simulink model "MySuspKnC_RTW"  (Simulink 9.3)
settings: Solver=ode1  StartTime=0.0  StopTime=inf  FixedStep=0.001  RelTol=1e-3
PreLoadFcn:
  | vehicle = 'Car'; if ~length(which('cmself')), cmenv; end
  | MySuspKnC_RTW_bus
InitFcn:
  | vehicle = 'Car'; if ~length(which('cmself')), cmenv; end
  | MySuspKnC_RTW_bus
Description:
  | CarMaker Plug-in Model Target
settings Model: Creator=ml  LastModifiedBy=ml
settings DataIOCC: SaveFormat=Dataset  SignalLoggingSaveFormat=Dataset  ReturnWorkspaceOutputs=on
settings OptimizationCC: LifeSpan=auto
settings DebuggingCC: UnderspecifiedInitializationDetection=Simplified  MergeDetectMultiDrivingBlocksExec=error  FcnCallInpInsideContextMsg=error  SFUnexpectedBacktrackingDiag=error  SFNoUnconditionalDefaultTransitionDiag=error  SFExecutionAtInitializationDiag=warning  ArithmeticOperatorsInVariantConditions=error
settings HardwareCC: ProdBitPerPointer=64  ProdBitPerSizeT=64  ProdBitPerPtrDiffT=64  ProdLargestAtomicFloat=Float  ProdIntDivRoundTo=Zero  ProdEndianess=LittleEndian  ProdWordSize=64  ProdHWDeviceType=Intel->x86-64 (Windows64)
settings ModelReferenceCC: PropagateSignalLabelsOutOfModel=on
settings SFSimCC: SimUseLocalCustomCode=on
settings RTWCC: SystemTargetFile=CarMaker.tlc  TemplateMakefile=CarMaker_unix-win64.tmf  Description=CarMaker Plug-in Model Target  RTWUseLocalCustomCode=on
settings CodeAppCC: MaxIdLength=127  StateflowObjectComments=off
settings STFCustomTargetCC: TargetLangStandard=C99 (ISO)  CombineOutputUpdateFcns=on  MultiInstanceERTCode=on  CodeInterfacePackaging=Reusable function  GRTInterface=off  GenerateAllocFcn=on  SystemTargetFile=CarMaker.tlc
settings GRTTargetCC: TargetLangStandard=C99 (ISO)  ParMdlRefBuildCompliant=off  CompOptLevelCompliant=off  ConcurrentExecutionCompliant=off  CombineOutputUpdateFcns=on  MatFileLogging=off  MultiInstanceERTCode=on  CodeInterfacePackaging=Reusable function  CPPClassGenCompliant=off  GRTInterface=off  GenerateAllocFcn=on  UseToolchainInfoCompliant=off  RTWCAPISignals=on  RTWCAPIParams=on
settings CustomProperty: DataType=string
settings EnumStrPairs: String=Car
settings ConfigComp: CovMetricSettings=dwe  CovHtmlReporting=off  CovSaveCumulativeToWorkspaceVar=off  CovSaveSingleToWorkspaceVar=off  CovExternalEMLEnable=on

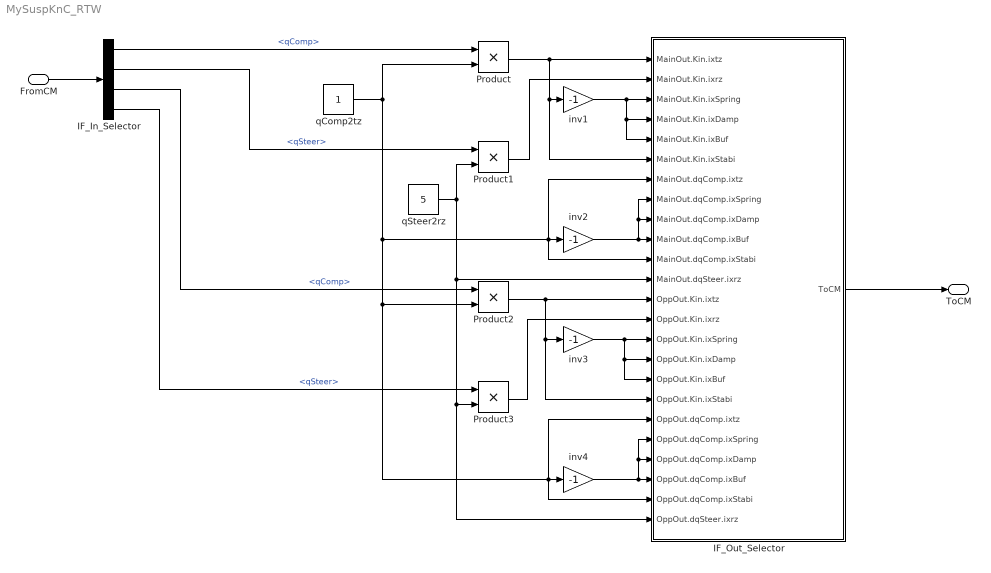
== system MySuspKnC_RTW ==
  FromCM : Inport  OutDataTypeStr=Bus: cmSuspKnCIn
  IF_In_Selector : BusSelector  OutputSignals=MainIn.qComp,MainIn.qSteer,OppIn.qComp,OppIn.qSteer
  IF_Out_Selector : Subsystem  mask(Signal Selection){}
      mask help: Signal Selection Block
      settings: OpenFcn=cmSignalSelect('SignalSelection_CB',gcb)
  Product{,1..3} (4 alike) : Product
  inv{1..4} (4 alike) : Gain  Gain=-1
  qComp2tz : Constant
  qSteer2rz : Constant  Value=5
  ToCM : Outport  OutDataTypeStr=Bus: cmSuspKnCOut
  wires:
  FromCM/1 -> IF_In_Selector/1
  IF_Out_Selector/1(ToCM) -> ToCM/1
  qSteer2rz/1 -> Product1/2, IF_Out_Selector/12(MainOut.dqSteer.ixrz), IF_Out_Selector/24(OppOut.dqSteer.ixrz), Product3/2
  IF_In_Selector/1 -> Product/1  "<qComp>"
  IF_In_Selector/2 -> Product1/1  "<qSteer>"
  qComp2tz/1 -> Product/2, IF_Out_Selector/7(MainOut.dqComp.ixtz), inv2/1, IF_Out_Selector/11(MainOut.dqComp.ixStabi), IF_Out_Selector/19(OppOut.dqComp.ixtz), IF_Out_Selector/23(OppOut.dqComp.ixStabi), inv4/1, Product2/2
  Product/1 -> IF_Out_Selector/6(MainOut.Kin.ixStabi), inv1/1, IF_Out_Selector/1(MainOut.Kin.ixtz)
  Product1/1 -> IF_Out_Selector/2(MainOut.Kin.ixrz)
  inv2/1 -> IF_Out_Selector/9(MainOut.dqComp.ixDamp), IF_Out_Selector/8(MainOut.dqComp.ixSpring), IF_Out_Selector/10(MainOut.dqComp.ixBuf)
  inv1/1 -> IF_Out_Selector/3(MainOut.Kin.ixSpring), IF_Out_Selector/4(MainOut.Kin.ixDamp), IF_Out_Selector/5(MainOut.Kin.ixBuf)
  IF_In_Selector/3 -> Product2/1  "<qComp>"
  IF_In_Selector/4 -> Product3/1  "<qSteer>"
  inv3/1 -> IF_Out_Selector/17(OppOut.Kin.ixBuf), IF_Out_Selector/16(OppOut.Kin.ixDamp), IF_Out_Selector/15(OppOut.Kin.ixSpring)
  Product2/1 -> IF_Out_Selector/18(OppOut.Kin.ixStabi), inv3/1, IF_Out_Selector/13(OppOut.Kin.ixtz)
  Product3/1 -> IF_Out_Selector/14(OppOut.Kin.ixrz)
  inv4/1 -> IF_Out_Selector/20(OppOut.dqComp.ixSpring), IF_Out_Selector/21(OppOut.dqComp.ixDamp), IF_Out_Selector/22(OppOut.dqComp.ixBuf)

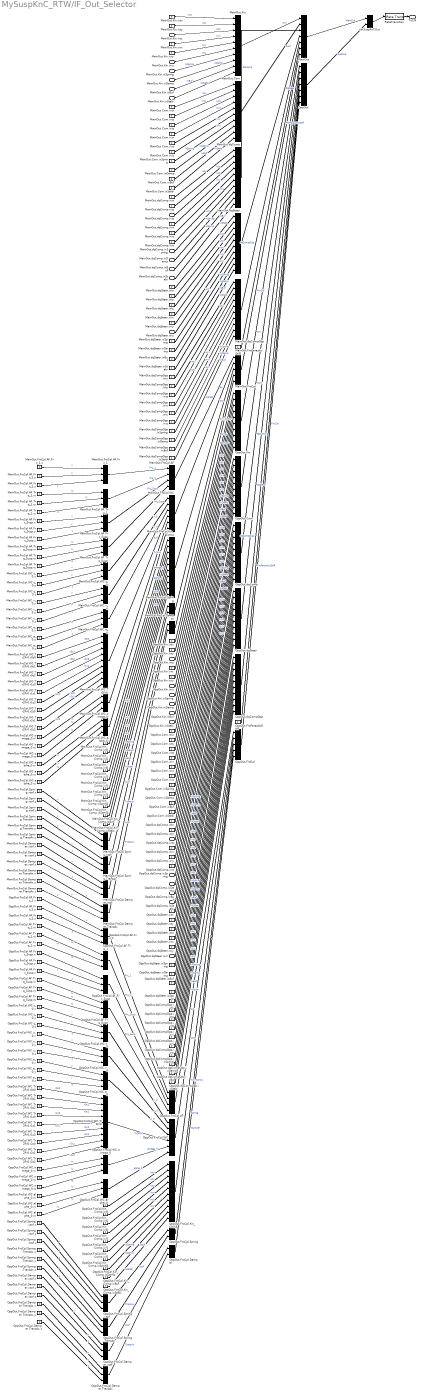
== system MySuspKnC_RTW/IF_Out_Selector ==
  MainOut.Kin.ixtz : Inport
  MainOut.Kin.ixrz : Inport  Port=2
  MainOut.Kin.ixSpring : Inport  Port=3
  MainOut.Kin.ixDamp : Inport  Port=4
  MainOut.Kin.ixBuf : Inport  Port=5
  MainOut.Kin.ixStabi : Inport  Port=6
  MainOut.dqComp.ixtz : Inport  Port=7
  MainOut.dqComp.ixSpring : Inport  Port=8
  MainOut.dqComp.ixDamp : Inport  Port=9
  MainOut.dqComp.ixBuf : Inport  Port=10
  MainOut.dqComp.ixStabi : Inport  Port=11
  MainOut.dqSteer.ixrz : Inport  Port=12
  OppOut.Kin.ixtz : Inport  Port=13
  OppOut.Kin.ixrz : Inport  Port=14
  OppOut.Kin.ixSpring : Inport  Port=15
  OppOut.Kin.ixDamp : Inport  Port=16
  OppOut.Kin.ixBuf : Inport  Port=17
  OppOut.Kin.ixStabi : Inport  Port=18
  OppOut.dqComp.ixtz : Inport  Port=19
  OppOut.dqComp.ixSpring : Inport  Port=20
  OppOut.dqComp.ixDamp : Inport  Port=21
  OppOut.dqComp.ixBuf : Inport  Port=22
  OppOut.dqComp.ixStabi : Inport  Port=23
  OppOut.dqSteer.ixrz : Inport  Port=24
  MainOut : BusCreator  Inputs=7
  MainOut.Com : BusCreator  Inputs=10
  MainOut.Com.ixBuf : Constant  Value=0
  MainOut.Com.ixDamp : Constant  Value=0
  MainOut.Com.ixSpring : Constant  Value=0
  MainOut.Com.ixStabi : Constant  Value=0
  MainOut.Com.ixrx : Constant  Value=0
  MainOut.Com.ixry : Constant  Value=0
  MainOut.Com.ixrz : Constant  Value=0
  MainOut.Com.ixtx : Constant  Value=0
  MainOut.Com.ixty : Constant  Value=0
  MainOut.Com.ixtz : Constant  Value=0
  MainOut.FrcCpl : BusCreator  Inputs=5
  MainOut.FrcCpl.AF : BusCreator  Inputs=4
  MainOut.FrcCpl.AF.Frc_1 : BusCreator  Inputs=3
  MainOut.FrcCpl.AF.Frc_1.x : Constant  Value=0
  MainOut.FrcCpl.AF.Frc_1.y : Constant  Value=0
  MainOut.FrcCpl.AF.Frc_1.z : Constant  Value=0
  MainOut.FrcCpl.AF.Frc_Susp : BusCreator  Inputs=3
  MainOut.FrcCpl.AF.Frc_Susp.x : Constant  Value=0
  MainOut.FrcCpl.AF.Frc_Susp.y : Constant  Value=0
  MainOut.FrcCpl.AF.Frc_Susp.z : Constant  Value=0
  MainOut.FrcCpl.AF.Trq_1 : BusCreator  Inputs=3
  MainOut.FrcCpl.AF.Trq_1.rx : Constant  Value=0
  MainOut.FrcCpl.AF.Trq_1.ry : Constant  Value=0
  MainOut.FrcCpl.AF.Trq_1.rz : Constant  Value=0
  MainOut.FrcCpl.AF.Trq_Susp : BusCreator  Inputs=3
  MainOut.FrcCpl.AF.Trq_Susp.rx : Constant  Value=0
  MainOut.FrcCpl.AF.Trq_Susp.ry : Constant  Value=0
  MainOut.FrcCpl.AF.Trq_Susp.rz : Constant  Value=0
  MainOut.FrcCpl.Damper : BusCreator  Inputs=2
  MainOut.FrcCpl.Damper.TransAx : BusCreator  Inputs=3
  MainOut.FrcCpl.Damper.TransAx.x : Constant  Value=0
  MainOut.FrcCpl.Damper.TransAx.y : Constant  Value=0
  MainOut.FrcCpl.Damper.TransAx.z : Constant  Value=0
  MainOut.FrcCpl.Damper.xtof : BusCreator  Inputs=3
  MainOut.FrcCpl.Damper.xtof.x : Constant  Value=0
  MainOut.FrcCpl.Damper.xtof.y : Constant  Value=0
  MainOut.FrcCpl.Damper.xtof.z : Constant  Value=0
  MainOut.FrcCpl.Kin_Comp : BusCreator  Inputs=10
  MainOut.FrcCpl.Kin_Comp.ixBuf : Constant  Value=0
  MainOut.FrcCpl.Kin_Comp.ixDamp : Constant  Value=0
  MainOut.FrcCpl.Kin_Comp.ixSpring : Constant  Value=0
  MainOut.FrcCpl.Kin_Comp.ixStabi : Constant  Value=0
  MainOut.FrcCpl.Kin_Comp.ixrx : Constant  Value=0
  MainOut.FrcCpl.Kin_Comp.ixry : Constant  Value=0
  MainOut.FrcCpl.Kin_Comp.ixrz : Constant  Value=0
  MainOut.FrcCpl.Kin_Comp.ixtx : Constant  Value=0
  MainOut.FrcCpl.Kin_Comp.ixty : Constant  Value=0
  MainOut.FrcCpl.Kin_Comp.ixtz : Constant  Value=0
  MainOut.FrcCpl.Spring : BusCreator  Inputs=2
  MainOut.FrcCpl.Spring.TransAx : BusCreator  Inputs=3
  MainOut.FrcCpl.Spring.TransAx.x : Constant  Value=0
  MainOut.FrcCpl.Spring.TransAx.y : Constant  Value=0
  MainOut.FrcCpl.Spring.TransAx.z : Constant  Value=0
  MainOut.FrcCpl.Spring.xtof : BusCreator  Inputs=3
  MainOut.FrcCpl.Spring.xtof.x : Constant  Value=0
  MainOut.FrcCpl.Spring.xtof.y : Constant  Value=0
  MainOut.FrcCpl.Spring.xtof.z : Constant  Value=0
  MainOut.FrcCpl.WC : BusCreator  Inputs=6
  MainOut.FrcCpl.WC.Tr2Fr0 : BusCreator  Inputs=9
  MainOut.FrcCpl.WC.Tr2Fr0.r0c0 : Constant  Value=0
  MainOut.FrcCpl.WC.Tr2Fr0.r0c1 : Constant  Value=0
  MainOut.FrcCpl.WC.Tr2Fr0.r0c2 : Constant  Value=0
  MainOut.FrcCpl.WC.Tr2Fr0.r1c0 : Constant  Value=0
  MainOut.FrcCpl.WC.Tr2Fr0.r1c1 : Constant  Value=0
  MainOut.FrcCpl.WC.Tr2Fr0.r1c2 : Constant  Value=0
  MainOut.FrcCpl.WC.Tr2Fr0.r2c0 : Constant  Value=0
  MainOut.FrcCpl.WC.Tr2Fr0.r2c1 : Constant  Value=0
  MainOut.FrcCpl.WC.Tr2Fr0.r2c2 : Constant  Value=0
  MainOut.FrcCpl.WC.a_0 : BusCreator  Inputs=3
  MainOut.FrcCpl.WC.a_0.x : Constant  Value=0
  MainOut.FrcCpl.WC.a_0.y : Constant  Value=0
  MainOut.FrcCpl.WC.a_0.z : Constant  Value=0
  MainOut.FrcCpl.WC.alpha_0 : BusCreator  Inputs=3
  MainOut.FrcCpl.WC.alpha_0.rx : Constant  Value=0
  MainOut.FrcCpl.WC.alpha_0.ry : Constant  Value=0
  MainOut.FrcCpl.WC.alpha_0.rz : Constant  Value=0
  MainOut.FrcCpl.WC.omega_0 : BusCreator  Inputs=3
  MainOut.FrcCpl.WC.omega_0.rx : Constant  Value=0
  MainOut.FrcCpl.WC.omega_0.ry : Constant  Value=0
  MainOut.FrcCpl.WC.omega_0.rz : Constant  Value=0
  MainOut.FrcCpl.WC.t_0 : BusCreator  Inputs=3
  MainOut.FrcCpl.WC.t_0.x : Constant  Value=0
  MainOut.FrcCpl.WC.t_0.y : Constant  Value=0
  MainOut.FrcCpl.WC.t_0.z : Constant  Value=0
  MainOut.FrcCpl.WC.v_0 : BusCreator  Inputs=3
  MainOut.FrcCpl.WC.v_0.x : Constant  Value=0
  MainOut.FrcCpl.WC.v_0.y : Constant  Value=0
  MainOut.FrcCpl.WC.v_0.z : Constant  Value=0
  MainOut.FrcParasiticStiff : Constant  Value=0
  MainOut.Kin : BusCreator  Inputs=10
  MainOut.Kin.ixrx : Constant  Value=0
  MainOut.Kin.ixry : Constant  Value=0
  MainOut.Kin.ixtx : Constant  Value=0
  MainOut.Kin.ixty : Constant  Value=0
  MainOut.dqComp : BusCreator  Inputs=10
  MainOut.dqComp.ixrx : Constant  Value=0
  MainOut.dqComp.ixry : Constant  Value=0
  MainOut.dqComp.ixrz : Constant  Value=0
  MainOut.dqComp.ixtx : Constant  Value=0
  MainOut.dqComp.ixty : Constant  Value=0
  MainOut.dqCompOpp : BusCreator  Inputs=10
  MainOut.dqCompOpp.ixBuf : Constant  Value=0
  MainOut.dqCompOpp.ixDamp : Constant  Value=0
  MainOut.dqCompOpp.ixSpring : Constant  Value=0
  MainOut.dqCompOpp.ixStabi : Constant  Value=0
  MainOut.dqCompOpp.ixrx : Constant  Value=0
  MainOut.dqCompOpp.ixry : Constant  Value=0
  MainOut.dqCompOpp.ixrz : Constant  Value=0
  MainOut.dqCompOpp.ixtx : Constant  Value=0
  MainOut.dqCompOpp.ixty : Constant  Value=0
  MainOut.dqCompOpp.ixtz : Constant  Value=0
  MainOut.dqSteer : BusCreator  Inputs=10
  MainOut.dqSteer.ixBuf : Constant  Value=0
  MainOut.dqSteer.ixDamp : Constant  Value=0
  MainOut.dqSteer.ixSpring : Constant  Value=0
  MainOut.dqSteer.ixStabi : Constant  Value=0
  MainOut.dqSteer.ixrx : Constant  Value=0
  MainOut.dqSteer.ixry : Constant  Value=0
  MainOut.dqSteer.ixtx : Constant  Value=0
  MainOut.dqSteer.ixty : Constant  Value=0
  MainOut.dqSteer.ixtz : Constant  Value=0
  OppOut : BusCreator  Inputs=7
  OppOut.Com : BusCreator  Inputs=10
  OppOut.Com.ixBuf : Constant  Value=0
  OppOut.Com.ixDamp : Constant  Value=0
  OppOut.Com.ixSpring : Constant  Value=0
  OppOut.Com.ixStabi : Constant  Value=0
  OppOut.Com.ixrx : Constant  Value=0
  OppOut.Com.ixry : Constant  Value=0
  OppOut.Com.ixrz : Constant  Value=0
  OppOut.Com.ixtx : Constant  Value=0
  OppOut.Com.ixty : Constant  Value=0
  OppOut.Com.ixtz : Constant  Value=0
  OppOut.FrcCpl : BusCreator  Inputs=5
  OppOut.FrcCpl.AF : BusCreator  Inputs=4
  OppOut.FrcCpl.AF.Frc_1 : BusCreator  Inputs=3
  OppOut.FrcCpl.AF.Frc_1.x : Constant  Value=0
  OppOut.FrcCpl.AF.Frc_1.y : Constant  Value=0
  OppOut.FrcCpl.AF.Frc_1.z : Constant  Value=0
  OppOut.FrcCpl.AF.Frc_Susp : BusCreator  Inputs=3
  OppOut.FrcCpl.AF.Frc_Susp.x : Constant  Value=0
  OppOut.FrcCpl.AF.Frc_Susp.y : Constant  Value=0
  OppOut.FrcCpl.AF.Frc_Susp.z : Constant  Value=0
  OppOut.FrcCpl.AF.Trq_1 : BusCreator  Inputs=3
  OppOut.FrcCpl.AF.Trq_1.rx : Constant  Value=0
  OppOut.FrcCpl.AF.Trq_1.ry : Constant  Value=0
  OppOut.FrcCpl.AF.Trq_1.rz : Constant  Value=0
  OppOut.FrcCpl.AF.Trq_Susp : BusCreator  Inputs=3
  OppOut.FrcCpl.AF.Trq_Susp.rx : Constant  Value=0
  OppOut.FrcCpl.AF.Trq_Susp.ry : Constant  Value=0
  OppOut.FrcCpl.AF.Trq_Susp.rz : Constant  Value=0
  OppOut.FrcCpl.Damper : BusCreator  Inputs=2
  OppOut.FrcCpl.Damper.TransAx : BusCreator  Inputs=3
  OppOut.FrcCpl.Damper.TransAx.x : Constant  Value=0
  OppOut.FrcCpl.Damper.TransAx.y : Constant  Value=0
  OppOut.FrcCpl.Damper.TransAx.z : Constant  Value=0
  OppOut.FrcCpl.Damper.xtof : BusCreator  Inputs=3
  OppOut.FrcCpl.Damper.xtof.x : Constant  Value=0
  OppOut.FrcCpl.Damper.xtof.y : Constant  Value=0
  OppOut.FrcCpl.Damper.xtof.z : Constant  Value=0
  OppOut.FrcCpl.Kin_Comp : BusCreator  Inputs=10
  OppOut.FrcCpl.Kin_Comp.ixBuf : Constant  Value=0
  OppOut.FrcCpl.Kin_Comp.ixDamp : Constant  Value=0
  OppOut.FrcCpl.Kin_Comp.ixSpring : Constant  Value=0
  OppOut.FrcCpl.Kin_Comp.ixStabi : Constant  Value=0
  OppOut.FrcCpl.Kin_Comp.ixrx : Constant  Value=0
  OppOut.FrcCpl.Kin_Comp.ixry : Constant  Value=0
  OppOut.FrcCpl.Kin_Comp.ixrz : Constant  Value=0
  OppOut.FrcCpl.Kin_Comp.ixtx : Constant  Value=0
  OppOut.FrcCpl.Kin_Comp.ixty : Constant  Value=0
  OppOut.FrcCpl.Kin_Comp.ixtz : Constant  Value=0
  OppOut.FrcCpl.Spring : BusCreator  Inputs=2
  OppOut.FrcCpl.Spring.TransAx : BusCreator  Inputs=3
  OppOut.FrcCpl.Spring.TransAx.x : Constant  Value=0
  OppOut.FrcCpl.Spring.TransAx.y : Constant  Value=0
  OppOut.FrcCpl.Spring.TransAx.z : Constant  Value=0
  OppOut.FrcCpl.Spring.xtof : BusCreator  Inputs=3
  OppOut.FrcCpl.Spring.xtof.x : Constant  Value=0
  OppOut.FrcCpl.Spring.xtof.y : Constant  Value=0
  OppOut.FrcCpl.Spring.xtof.z : Constant  Value=0
  OppOut.FrcCpl.WC : BusCreator  Inputs=6
  OppOut.FrcCpl.WC.Tr2Fr0 : BusCreator  Inputs=9
  OppOut.FrcCpl.WC.Tr2Fr0.r0c0 : Constant  Value=0
  OppOut.FrcCpl.WC.Tr2Fr0.r0c1 : Constant  Value=0
  OppOut.FrcCpl.WC.Tr2Fr0.r0c2 : Constant  Value=0
  OppOut.FrcCpl.WC.Tr2Fr0.r1c0 : Constant  Value=0
  OppOut.FrcCpl.WC.Tr2Fr0.r1c1 : Constant  Value=0
  OppOut.FrcCpl.WC.Tr2Fr0.r1c2 : Constant  Value=0
  OppOut.FrcCpl.WC.Tr2Fr0.r2c0 : Constant  Value=0
  OppOut.FrcCpl.WC.Tr2Fr0.r2c1 : Constant  Value=0
  OppOut.FrcCpl.WC.Tr2Fr0.r2c2 : Constant  Value=0
  OppOut.FrcCpl.WC.a_0 : BusCreator  Inputs=3
  OppOut.FrcCpl.WC.a_0.x : Constant  Value=0
  OppOut.FrcCpl.WC.a_0.y : Constant  Value=0
  OppOut.FrcCpl.WC.a_0.z : Constant  Value=0
  OppOut.FrcCpl.WC.alpha_0 : BusCreator  Inputs=3
  OppOut.FrcCpl.WC.alpha_0.rx : Constant  Value=0
  OppOut.FrcCpl.WC.alpha_0.ry : Constant  Value=0
  OppOut.FrcCpl.WC.alpha_0.rz : Constant  Value=0
  OppOut.FrcCpl.WC.omega_0 : BusCreator  Inputs=3
  OppOut.FrcCpl.WC.omega_0.rx : Constant  Value=0
  OppOut.FrcCpl.WC.omega_0.ry : Constant  Value=0
  OppOut.FrcCpl.WC.omega_0.rz : Constant  Value=0
  OppOut.FrcCpl.WC.t_0 : BusCreator  Inputs=3
  OppOut.FrcCpl.WC.t_0.x : Constant  Value=0
  OppOut.FrcCpl.WC.t_0.y : Constant  Value=0
  OppOut.FrcCpl.WC.t_0.z : Constant  Value=0
  OppOut.FrcCpl.WC.v_0 : BusCreator  Inputs=3
  OppOut.FrcCpl.WC.v_0.x : Constant  Value=0
  OppOut.FrcCpl.WC.v_0.y : Constant  Value=0
  OppOut.FrcCpl.WC.v_0.z : Constant  Value=0
  OppOut.FrcParasiticStiff : Constant  Value=0
  OppOut.Kin : BusCreator  Inputs=10
  OppOut.Kin.ixrx : Constant  Value=0
  OppOut.Kin.ixry : Constant  Value=0
  OppOut.Kin.ixtx : Constant  Value=0
  OppOut.Kin.ixty : Constant  Value=0
  OppOut.dqComp : BusCreator  Inputs=10
  OppOut.dqComp.ixrx : Constant  Value=0
  OppOut.dqComp.ixry : Constant  Value=0
  OppOut.dqComp.ixrz : Constant  Value=0
  OppOut.dqComp.ixtx : Constant  Value=0
  OppOut.dqComp.ixty : Constant  Value=0
  OppOut.dqCompOpp : BusCreator  Inputs=10
  OppOut.dqCompOpp.ixBuf : Constant  Value=0
  OppOut.dqCompOpp.ixDamp : Constant  Value=0
  OppOut.dqCompOpp.ixSpring : Constant  Value=0
  OppOut.dqCompOpp.ixStabi : Constant  Value=0
  OppOut.dqCompOpp.ixrx : Constant  Value=0
  OppOut.dqCompOpp.ixry : Constant  Value=0
  OppOut.dqCompOpp.ixrz : Constant  Value=0
  OppOut.dqCompOpp.ixtx : Constant  Value=0
  OppOut.dqCompOpp.ixty : Constant  Value=0
  OppOut.dqCompOpp.ixtz : Constant  Value=0
  OppOut.dqSteer : BusCreator  Inputs=10
  OppOut.dqSteer.ixBuf : Constant  Value=0
  OppOut.dqSteer.ixDamp : Constant  Value=0
  OppOut.dqSteer.ixSpring : Constant  Value=0
  OppOut.dqSteer.ixStabi : Constant  Value=0
  OppOut.dqSteer.ixrx : Constant  Value=0
  OppOut.dqSteer.ixry : Constant  Value=0
  OppOut.dqSteer.ixtx : Constant  Value=0
  OppOut.dqSteer.ixty : Constant  Value=0
  OppOut.dqSteer.ixtz : Constant  Value=0
  RateTransition : RateTransition  OutPortSampleTime=str2num(get_param(bdroot,'FixedStep'))
  cmSuspKnCOut : BusCreator  Inputs=2
  ToCM : Outport
  wires:
  RateTransition/1 -> ToCM/1
  cmSuspKnCOut/1 -> RateTransition/1
  MainOut/1 -> cmSuspKnCOut/1  "MainOut"
  MainOut.Kin/1 -> MainOut/1  "Kin"
  MainOut.Com/1 -> MainOut/2  "Com"
  MainOut.Com.ixtx/1 -> MainOut.Com/1  "ixtx"
  MainOut.Com.ixty/1 -> MainOut.Com/2  "ixty"
  MainOut.Com.ixtz/1 -> MainOut.Com/3  "ixtz"
  MainOut.Com.ixrx/1 -> MainOut.Com/4  "ixrx"
  MainOut.Com.ixry/1 -> MainOut.Com/5  "ixry"
  MainOut.Com.ixrz/1 -> MainOut.Com/6  "ixrz"
  MainOut.Com.ixSpring/1 -> MainOut.Com/7  "ixSpring"
  MainOut.Com.ixDamp/1 -> MainOut.Com/8  "ixDamp"
  MainOut.Com.ixBuf/1 -> MainOut.Com/9  "ixBuf"
  MainOut.Com.ixStabi/1 -> MainOut.Com/10  "ixStabi"
  MainOut.dqComp/1 -> MainOut/3  "dqComp"
  MainOut.dqComp.ixtx/1 -> MainOut.dqComp/1  "ixtx"
  MainOut.dqComp.ixty/1 -> MainOut.dqComp/2  "ixty"
  MainOut.dqComp.ixrx/1 -> MainOut.dqComp/4  "ixrx"
  MainOut.dqComp.ixry/1 -> MainOut.dqComp/5  "ixry"
  MainOut.dqComp.ixrz/1 -> MainOut.dqComp/6  "ixrz"
  MainOut.dqSteer/1 -> MainOut/4  "dqSteer"
  MainOut.dqSteer.ixtx/1 -> MainOut.dqSteer/1  "ixtx"
  MainOut.dqSteer.ixty/1 -> MainOut.dqSteer/2  "ixty"
  MainOut.dqSteer.ixtz/1 -> MainOut.dqSteer/3  "ixtz"
  MainOut.dqSteer.ixrx/1 -> MainOut.dqSteer/4  "ixrx"
  MainOut.dqSteer.ixry/1 -> MainOut.dqSteer/5  "ixry"
  MainOut.dqSteer.ixSpring/1 -> MainOut.dqSteer/7  "ixSpring"
  MainOut.dqSteer.ixDamp/1 -> MainOut.dqSteer/8  "ixDamp"
  MainOut.dqSteer.ixBuf/1 -> MainOut.dqSteer/9  "ixBuf"
  MainOut.dqSteer.ixStabi/1 -> MainOut.dqSteer/10  "ixStabi"
  MainOut.dqCompOpp/1 -> MainOut/5  "dqCompOpp"
  MainOut.dqCompOpp.ixtx/1 -> MainOut.dqCompOpp/1  "ixtx"
  MainOut.dqCompOpp.ixty/1 -> MainOut.dqCompOpp/2  "ixty"
  MainOut.dqCompOpp.ixtz/1 -> MainOut.dqCompOpp/3  "ixtz"
  MainOut.dqCompOpp.ixrx/1 -> MainOut.dqCompOpp/4  "ixrx"
  MainOut.dqCompOpp.ixry/1 -> MainOut.dqCompOpp/5  "ixry"
  MainOut.dqCompOpp.ixrz/1 -> MainOut.dqCompOpp/6  "ixrz"
  MainOut.dqCompOpp.ixSpring/1 -> MainOut.dqCompOpp/7  "ixSpring"
  MainOut.dqCompOpp.ixDamp/1 -> MainOut.dqCompOpp/8  "ixDamp"
  MainOut.dqCompOpp.ixBuf/1 -> MainOut.dqCompOpp/9  "ixBuf"
  MainOut.dqCompOpp.ixStabi/1 -> MainOut.dqCompOpp/10  "ixStabi"
  MainOut.FrcParasiticStiff/1 -> MainOut/6  "FrcParasiticStiff"
  MainOut.FrcCpl/1 -> MainOut/7  "FrcCpl"
  MainOut.FrcCpl.AF/1 -> MainOut.FrcCpl/1  "AF"
  MainOut.FrcCpl.AF.Frc_1/1 -> MainOut.FrcCpl.AF/1  "Frc_1"
  MainOut.FrcCpl.AF.Frc_1.x/1 -> MainOut.FrcCpl.AF.Frc_1/1  "x"
  MainOut.FrcCpl.AF.Frc_1.y/1 -> MainOut.FrcCpl.AF.Frc_1/2  "y"
  MainOut.FrcCpl.AF.Frc_1.z/1 -> MainOut.FrcCpl.AF.Frc_1/3  "z"
  MainOut.FrcCpl.AF.Trq_1/1 -> MainOut.FrcCpl.AF/2  "Trq_1"
  MainOut.FrcCpl.AF.Trq_1.rx/1 -> MainOut.FrcCpl.AF.Trq_1/1  "rx"
  MainOut.FrcCpl.AF.Trq_1.ry/1 -> MainOut.FrcCpl.AF.Trq_1/2  "ry"
  MainOut.FrcCpl.AF.Trq_1.rz/1 -> MainOut.FrcCpl.AF.Trq_1/3  "rz"
  MainOut.FrcCpl.AF.Frc_Susp/1 -> MainOut.FrcCpl.AF/3  "Frc_Susp"
  MainOut.FrcCpl.AF.Frc_Susp.x/1 -> MainOut.FrcCpl.AF.Frc_Susp/1  "x"
  MainOut.FrcCpl.AF.Frc_Susp.y/1 -> MainOut.FrcCpl.AF.Frc_Susp/2  "y"
  MainOut.FrcCpl.AF.Frc_Susp.z/1 -> MainOut.FrcCpl.AF.Frc_Susp/3  "z"
  MainOut.FrcCpl.AF.Trq_Susp/1 -> MainOut.FrcCpl.AF/4  "Trq_Susp"
  MainOut.FrcCpl.AF.Trq_Susp.rx/1 -> MainOut.FrcCpl.AF.Trq_Susp/1  "rx"
  MainOut.FrcCpl.AF.Trq_Susp.ry/1 -> MainOut.FrcCpl.AF.Trq_Susp/2  "ry"
  MainOut.FrcCpl.AF.Trq_Susp.rz/1 -> MainOut.FrcCpl.AF.Trq_Susp/3  "rz"
  MainOut.FrcCpl.WC/1 -> MainOut.FrcCpl/2  "WC"
  MainOut.FrcCpl.WC.t_0/1 -> MainOut.FrcCpl.WC/1  "t_0"
  MainOut.FrcCpl.WC.t_0.x/1 -> MainOut.FrcCpl.WC.t_0/1  "x"
  MainOut.FrcCpl.WC.t_0.y/1 -> MainOut.FrcCpl.WC.t_0/2  "y"
  MainOut.FrcCpl.WC.t_0.z/1 -> MainOut.FrcCpl.WC.t_0/3  "z"
  MainOut.FrcCpl.WC.v_0/1 -> MainOut.FrcCpl.WC/2  "v_0"
  MainOut.FrcCpl.WC.v_0.x/1 -> MainOut.FrcCpl.WC.v_0/1  "x"
  MainOut.FrcCpl.WC.v_0.y/1 -> MainOut.FrcCpl.WC.v_0/2  "y"
  MainOut.FrcCpl.WC.v_0.z/1 -> MainOut.FrcCpl.WC.v_0/3  "z"
  MainOut.FrcCpl.WC.a_0/1 -> MainOut.FrcCpl.WC/3  "a_0"
  MainOut.FrcCpl.WC.a_0.x/1 -> MainOut.FrcCpl.WC.a_0/1  "x"
  MainOut.FrcCpl.WC.a_0.y/1 -> MainOut.FrcCpl.WC.a_0/2  "y"
  MainOut.FrcCpl.WC.a_0.z/1 -> MainOut.FrcCpl.WC.a_0/3  "z"
  MainOut.FrcCpl.WC.Tr2Fr0/1 -> MainOut.FrcCpl.WC/4  "Tr2Fr0"
  MainOut.FrcCpl.WC.Tr2Fr0.r0c0/1 -> MainOut.FrcCpl.WC.Tr2Fr0/1  "r0c0"
  MainOut.FrcCpl.WC.Tr2Fr0.r0c1/1 -> MainOut.FrcCpl.WC.Tr2Fr0/2  "r0c1"
  MainOut.FrcCpl.WC.Tr2Fr0.r0c2/1 -> MainOut.FrcCpl.WC.Tr2Fr0/3  "r0c2"
  MainOut.FrcCpl.WC.Tr2Fr0.r1c0/1 -> MainOut.FrcCpl.WC.Tr2Fr0/4  "r1c0"
  MainOut.FrcCpl.WC.Tr2Fr0.r1c1/1 -> MainOut.FrcCpl.WC.Tr2Fr0/5  "r1c1"
  MainOut.FrcCpl.WC.Tr2Fr0.r1c2/1 -> MainOut.FrcCpl.WC.Tr2Fr0/6  "r1c2"
  MainOut.FrcCpl.WC.Tr2Fr0.r2c0/1 -> MainOut.FrcCpl.WC.Tr2Fr0/7  "r2c0"
  MainOut.FrcCpl.WC.Tr2Fr0.r2c1/1 -> MainOut.FrcCpl.WC.Tr2Fr0/8  "r2c1"
  MainOut.FrcCpl.WC.Tr2Fr0.r2c2/1 -> MainOut.FrcCpl.WC.Tr2Fr0/9  "r2c2"
  MainOut.FrcCpl.WC.omega_0/1 -> MainOut.FrcCpl.WC/5  "omega_0"
  MainOut.FrcCpl.WC.omega_0.rx/1 -> MainOut.FrcCpl.WC.omega_0/1  "rx"
  MainOut.FrcCpl.WC.omega_0.ry/1 -> MainOut.FrcCpl.WC.omega_0/2  "ry"
  MainOut.FrcCpl.WC.omega_0.rz/1 -> MainOut.FrcCpl.WC.omega_0/3  "rz"
  MainOut.FrcCpl.WC.alpha_0/1 -> MainOut.FrcCpl.WC/6  "alpha_0"
  MainOut.FrcCpl.WC.alpha_0.rx/1 -> MainOut.FrcCpl.WC.alpha_0/1  "rx"
  MainOut.FrcCpl.WC.alpha_0.ry/1 -> MainOut.FrcCpl.WC.alpha_0/2  "ry"
  MainOut.FrcCpl.WC.alpha_0.rz/1 -> MainOut.FrcCpl.WC.alpha_0/3  "rz"
  MainOut.FrcCpl.Kin_Comp/1 -> MainOut.FrcCpl/3  "Kin_Comp"
  MainOut.FrcCpl.Kin_Comp.ixtx/1 -> MainOut.FrcCpl.Kin_Comp/1  "ixtx"
  MainOut.FrcCpl.Kin_Comp.ixty/1 -> MainOut.FrcCpl.Kin_Comp/2  "ixty"
  MainOut.FrcCpl.Kin_Comp.ixtz/1 -> MainOut.FrcCpl.Kin_Comp/3  "ixtz"
  MainOut.FrcCpl.Kin_Comp.ixrx/1 -> MainOut.FrcCpl.Kin_Comp/4  "ixrx"
  MainOut.FrcCpl.Kin_Comp.ixry/1 -> MainOut.FrcCpl.Kin_Comp/5  "ixry"
  MainOut.FrcCpl.Kin_Comp.ixrz/1 -> MainOut.FrcCpl.Kin_Comp/6  "ixrz"
  MainOut.FrcCpl.Kin_Comp.ixSpring/1 -> MainOut.FrcCpl.Kin_Comp/7  "ixSpring"
  MainOut.FrcCpl.Kin_Comp.ixDamp/1 -> MainOut.FrcCpl.Kin_Comp/8  "ixDamp"
  MainOut.FrcCpl.Kin_Comp.ixBuf/1 -> MainOut.FrcCpl.Kin_Comp/9  "ixBuf"
  MainOut.FrcCpl.Kin_Comp.ixStabi/1 -> MainOut.FrcCpl.Kin_Comp/10  "ixStabi"
  MainOut.FrcCpl.Spring/1 -> MainOut.FrcCpl/4  "Spring"
  MainOut.FrcCpl.Spring.xtof/1 -> MainOut.FrcCpl.Spring/1  "xtof"
  MainOut.FrcCpl.Spring.xtof.x/1 -> MainOut.FrcCpl.Spring.xtof/1  "x"
  MainOut.FrcCpl.Spring.xtof.y/1 -> MainOut.FrcCpl.Spring.xtof/2  "y"
  MainOut.FrcCpl.Spring.xtof.z/1 -> MainOut.FrcCpl.Spring.xtof/3  "z"
  MainOut.FrcCpl.Spring.TransAx/1 -> MainOut.FrcCpl.Spring/2  "TransAx"
  MainOut.FrcCpl.Spring.TransAx.x/1 -> MainOut.FrcCpl.Spring.TransAx/1  "x"
  MainOut.FrcCpl.Spring.TransAx.y/1 -> MainOut.FrcCpl.Spring.TransAx/2  "y"
  MainOut.FrcCpl.Spring.TransAx.z/1 -> MainOut.FrcCpl.Spring.TransAx/3  "z"
  MainOut.FrcCpl.Damper/1 -> MainOut.FrcCpl/5  "Damper"
  MainOut.FrcCpl.Damper.xtof/1 -> MainOut.FrcCpl.Damper/1  "xtof"
  MainOut.FrcCpl.Damper.xtof.x/1 -> MainOut.FrcCpl.Damper.xtof/1  "x"
  MainOut.FrcCpl.Damper.xtof.y/1 -> MainOut.FrcCpl.Damper.xtof/2  "y"
  MainOut.FrcCpl.Damper.xtof.z/1 -> MainOut.FrcCpl.Damper.xtof/3  "z"
  MainOut.FrcCpl.Damper.TransAx/1 -> MainOut.FrcCpl.Damper/2  "TransAx"
  MainOut.FrcCpl.Damper.TransAx.x/1 -> MainOut.FrcCpl.Damper.TransAx/1  "x"
  MainOut.FrcCpl.Damper.TransAx.y/1 -> MainOut.FrcCpl.Damper.TransAx/2  "y"
  MainOut.FrcCpl.Damper.TransAx.z/1 -> MainOut.FrcCpl.Damper.TransAx/3  "z"
  OppOut/1 -> cmSuspKnCOut/2  "OppOut"
  OppOut.Kin/1 -> OppOut/1  "Kin"
  OppOut.Kin.ixtx/1 -> OppOut.Kin/1  "ixtx"
  OppOut.Kin.ixty/1 -> OppOut.Kin/2  "ixty"
  OppOut.Kin.ixrx/1 -> OppOut.Kin/4  "ixrx"
  OppOut.Kin.ixry/1 -> OppOut.Kin/5  "ixry"
  OppOut.Com/1 -> OppOut/2  "Com"
  OppOut.Com.ixtx/1 -> OppOut.Com/1  "ixtx"
  OppOut.Com.ixty/1 -> OppOut.Com/2  "ixty"
  OppOut.Com.ixtz/1 -> OppOut.Com/3  "ixtz"
  OppOut.Com.ixrx/1 -> OppOut.Com/4  "ixrx"
  OppOut.Com.ixry/1 -> OppOut.Com/5  "ixry"
  OppOut.Com.ixrz/1 -> OppOut.Com/6  "ixrz"
  OppOut.Com.ixSpring/1 -> OppOut.Com/7  "ixSpring"
  OppOut.Com.ixDamp/1 -> OppOut.Com/8  "ixDamp"
  OppOut.Com.ixBuf/1 -> OppOut.Com/9  "ixBuf"
  OppOut.Com.ixStabi/1 -> OppOut.Com/10  "ixStabi"
  OppOut.dqComp/1 -> OppOut/3  "dqComp"
  OppOut.dqComp.ixtx/1 -> OppOut.dqComp/1  "ixtx"
  OppOut.dqComp.ixty/1 -> OppOut.dqComp/2  "ixty"
  OppOut.dqComp.ixrx/1 -> OppOut.dqComp/4  "ixrx"
  OppOut.dqComp.ixry/1 -> OppOut.dqComp/5  "ixry"
  OppOut.dqComp.ixrz/1 -> OppOut.dqComp/6  "ixrz"
  OppOut.dqSteer/1 -> OppOut/4  "dqSteer"
  OppOut.dqSteer.ixtx/1 -> OppOut.dqSteer/1  "ixtx"
  OppOut.dqSteer.ixty/1 -> OppOut.dqSteer/2  "ixty"
  OppOut.dqSteer.ixtz/1 -> OppOut.dqSteer/3  "ixtz"
  OppOut.dqSteer.ixrx/1 -> OppOut.dqSteer/4  "ixrx"
  OppOut.dqSteer.ixry/1 -> OppOut.dqSteer/5  "ixry"
  OppOut.dqSteer.ixSpring/1 -> OppOut.dqSteer/7  "ixSpring"
  OppOut.dqSteer.ixDamp/1 -> OppOut.dqSteer/8  "ixDamp"
  OppOut.dqSteer.ixBuf/1 -> OppOut.dqSteer/9  "ixBuf"
  OppOut.dqSteer.ixStabi/1 -> OppOut.dqSteer/10  "ixStabi"
  OppOut.dqCompOpp/1 -> OppOut/5  "dqCompOpp"
  OppOut.dqCompOpp.ixtx/1 -> OppOut.dqCompOpp/1  "ixtx"
  OppOut.dqCompOpp.ixty/1 -> OppOut.dqCompOpp/2  "ixty"
  OppOut.dqCompOpp.ixtz/1 -> OppOut.dqCompOpp/3  "ixtz"
  OppOut.dqCompOpp.ixrx/1 -> OppOut.dqCompOpp/4  "ixrx"
  OppOut.dqCompOpp.ixry/1 -> OppOut.dqCompOpp/5  "ixry"
  OppOut.dqCompOpp.ixrz/1 -> OppOut.dqCompOpp/6  "ixrz"
  OppOut.dqCompOpp.ixSpring/1 -> OppOut.dqCompOpp/7  "ixSpring"
  OppOut.dqCompOpp.ixDamp/1 -> OppOut.dqCompOpp/8  "ixDamp"
  OppOut.dqCompOpp.ixBuf/1 -> OppOut.dqCompOpp/9  "ixBuf"
  OppOut.dqCompOpp.ixStabi/1 -> OppOut.dqCompOpp/10  "ixStabi"
  OppOut.FrcParasiticStiff/1 -> OppOut/6  "FrcParasiticStiff"
  OppOut.FrcCpl/1 -> OppOut/7  "FrcCpl"
  OppOut.FrcCpl.AF/1 -> OppOut.FrcCpl/1  "AF"
  OppOut.FrcCpl.AF.Frc_1/1 -> OppOut.FrcCpl.AF/1  "Frc_1"
  OppOut.FrcCpl.AF.Frc_1.x/1 -> OppOut.FrcCpl.AF.Frc_1/1  "x"
  OppOut.FrcCpl.AF.Frc_1.y/1 -> OppOut.FrcCpl.AF.Frc_1/2  "y"
  OppOut.FrcCpl.AF.Frc_1.z/1 -> OppOut.FrcCpl.AF.Frc_1/3  "z"
  OppOut.FrcCpl.AF.Trq_1/1 -> OppOut.FrcCpl.AF/2  "Trq_1"
  OppOut.FrcCpl.AF.Trq_1.rx/1 -> OppOut.FrcCpl.AF.Trq_1/1  "rx"
  OppOut.FrcCpl.AF.Trq_1.ry/1 -> OppOut.FrcCpl.AF.Trq_1/2  "ry"
  OppOut.FrcCpl.AF.Trq_1.rz/1 -> OppOut.FrcCpl.AF.Trq_1/3  "rz"
  OppOut.FrcCpl.AF.Frc_Susp/1 -> OppOut.FrcCpl.AF/3  "Frc_Susp"
  OppOut.FrcCpl.AF.Frc_Susp.x/1 -> OppOut.FrcCpl.AF.Frc_Susp/1  "x"
  OppOut.FrcCpl.AF.Frc_Susp.y/1 -> OppOut.FrcCpl.AF.Frc_Susp/2  "y"
  OppOut.FrcCpl.AF.Frc_Susp.z/1 -> OppOut.FrcCpl.AF.Frc_Susp/3  "z"
  OppOut.FrcCpl.AF.Trq_Susp/1 -> OppOut.FrcCpl.AF/4  "Trq_Susp"
  OppOut.FrcCpl.AF.Trq_Susp.rx/1 -> OppOut.FrcCpl.AF.Trq_Susp/1  "rx"
  OppOut.FrcCpl.AF.Trq_Susp.ry/1 -> OppOut.FrcCpl.AF.Trq_Susp/2  "ry"
  OppOut.FrcCpl.AF.Trq_Susp.rz/1 -> OppOut.FrcCpl.AF.Trq_Susp/3  "rz"
  OppOut.FrcCpl.WC/1 -> OppOut.FrcCpl/2  "WC"
  OppOut.FrcCpl.WC.t_0/1 -> OppOut.FrcCpl.WC/1  "t_0"
  OppOut.FrcCpl.WC.t_0.x/1 -> OppOut.FrcCpl.WC.t_0/1  "x"
  OppOut.FrcCpl.WC.t_0.y/1 -> OppOut.FrcCpl.WC.t_0/2  "y"
  OppOut.FrcCpl.WC.t_0.z/1 -> OppOut.FrcCpl.WC.t_0/3  "z"
  OppOut.FrcCpl.WC.v_0/1 -> OppOut.FrcCpl.WC/2  "v_0"
  OppOut.FrcCpl.WC.v_0.x/1 -> OppOut.FrcCpl.WC.v_0/1  "x"
  OppOut.FrcCpl.WC.v_0.y/1 -> OppOut.FrcCpl.WC.v_0/2  "y"
  OppOut.FrcCpl.WC.v_0.z/1 -> OppOut.FrcCpl.WC.v_0/3  "z"
  OppOut.FrcCpl.WC.a_0/1 -> OppOut.FrcCpl.WC/3  "a_0"
  OppOut.FrcCpl.WC.a_0.x/1 -> OppOut.FrcCpl.WC.a_0/1  "x"
  OppOut.FrcCpl.WC.a_0.y/1 -> OppOut.FrcCpl.WC.a_0/2  "y"
  OppOut.FrcCpl.WC.a_0.z/1 -> OppOut.FrcCpl.WC.a_0/3  "z"
  OppOut.FrcCpl.WC.Tr2Fr0/1 -> OppOut.FrcCpl.WC/4  "Tr2Fr0"
  OppOut.FrcCpl.WC.Tr2Fr0.r0c0/1 -> OppOut.FrcCpl.WC.Tr2Fr0/1  "r0c0"
  OppOut.FrcCpl.WC.Tr2Fr0.r0c1/1 -> OppOut.FrcCpl.WC.Tr2Fr0/2  "r0c1"
  OppOut.FrcCpl.WC.Tr2Fr0.r0c2/1 -> OppOut.FrcCpl.WC.Tr2Fr0/3  "r0c2"
  OppOut.FrcCpl.WC.Tr2Fr0.r1c0/1 -> OppOut.FrcCpl.WC.Tr2Fr0/4  "r1c0"
  OppOut.FrcCpl.WC.Tr2Fr0.r1c1/1 -> OppOut.FrcCpl.WC.Tr2Fr0/5  "r1c1"
  OppOut.FrcCpl.WC.Tr2Fr0.r1c2/1 -> OppOut.FrcCpl.WC.Tr2Fr0/6  "r1c2"
  OppOut.FrcCpl.WC.Tr2Fr0.r2c0/1 -> OppOut.FrcCpl.WC.Tr2Fr0/7  "r2c0"
  OppOut.FrcCpl.WC.Tr2Fr0.r2c1/1 -> OppOut.FrcCpl.WC.Tr2Fr0/8  "r2c1"
  OppOut.FrcCpl.WC.Tr2Fr0.r2c2/1 -> OppOut.FrcCpl.WC.Tr2Fr0/9  "r2c2"
  OppOut.FrcCpl.WC.omega_0/1 -> OppOut.FrcCpl.WC/5  "omega_0"
  OppOut.FrcCpl.WC.omega_0.rx/1 -> OppOut.FrcCpl.WC.omega_0/1  "rx"
  OppOut.FrcCpl.WC.omega_0.ry/1 -> OppOut.FrcCpl.WC.omega_0/2  "ry"
  OppOut.FrcCpl.WC.omega_0.rz/1 -> OppOut.FrcCpl.WC.omega_0/3  "rz"
  OppOut.FrcCpl.WC.alpha_0/1 -> OppOut.FrcCpl.WC/6  "alpha_0"
  OppOut.FrcCpl.WC.alpha_0.rx/1 -> OppOut.FrcCpl.WC.alpha_0/1  "rx"
  OppOut.FrcCpl.WC.alpha_0.ry/1 -> OppOut.FrcCpl.WC.alpha_0/2  "ry"
  OppOut.FrcCpl.WC.alpha_0.rz/1 -> OppOut.FrcCpl.WC.alpha_0/3  "rz"
  OppOut.FrcCpl.Kin_Comp/1 -> OppOut.FrcCpl/3  "Kin_Comp"
  OppOut.FrcCpl.Kin_Comp.ixtx/1 -> OppOut.FrcCpl.Kin_Comp/1  "ixtx"
  OppOut.FrcCpl.Kin_Comp.ixty/1 -> OppOut.FrcCpl.Kin_Comp/2  "ixty"
  OppOut.FrcCpl.Kin_Comp.ixtz/1 -> OppOut.FrcCpl.Kin_Comp/3  "ixtz"
  OppOut.FrcCpl.Kin_Comp.ixrx/1 -> OppOut.FrcCpl.Kin_Comp/4  "ixrx"
  OppOut.FrcCpl.Kin_Comp.ixry/1 -> OppOut.FrcCpl.Kin_Comp/5  "ixry"
  OppOut.FrcCpl.Kin_Comp.ixrz/1 -> OppOut.FrcCpl.Kin_Comp/6  "ixrz"
  OppOut.FrcCpl.Kin_Comp.ixSpring/1 -> OppOut.FrcCpl.Kin_Comp/7  "ixSpring"
  OppOut.FrcCpl.Kin_Comp.ixDamp/1 -> OppOut.FrcCpl.Kin_Comp/8  "ixDamp"
  OppOut.FrcCpl.Kin_Comp.ixBuf/1 -> OppOut.FrcCpl.Kin_Comp/9  "ixBuf"
  OppOut.FrcCpl.Kin_Comp.ixStabi/1 -> OppOut.FrcCpl.Kin_Comp/10  "ixStabi"
  OppOut.FrcCpl.Spring/1 -> OppOut.FrcCpl/4  "Spring"
  OppOut.FrcCpl.Spring.xtof/1 -> OppOut.FrcCpl.Spring/1  "xtof"
  OppOut.FrcCpl.Spring.xtof.x/1 -> OppOut.FrcCpl.Spring.xtof/1  "x"
  OppOut.FrcCpl.Spring.xtof.y/1 -> OppOut.FrcCpl.Spring.xtof/2  "y"
  OppOut.FrcCpl.Spring.xtof.z/1 -> OppOut.FrcCpl.Spring.xtof/3  "z"
  OppOut.FrcCpl.Spring.TransAx/1 -> OppOut.FrcCpl.Spring/2  "TransAx"
  OppOut.FrcCpl.Spring.TransAx.x/1 -> OppOut.FrcCpl.Spring.TransAx/1  "x"
  OppOut.FrcCpl.Spring.TransAx.y/1 -> OppOut.FrcCpl.Spring.TransAx/2  "y"
  OppOut.FrcCpl.Spring.TransAx.z/1 -> OppOut.FrcCpl.Spring.TransAx/3  "z"
  OppOut.FrcCpl.Damper/1 -> OppOut.FrcCpl/5  "Damper"
  OppOut.FrcCpl.Damper.xtof/1 -> OppOut.FrcCpl.Damper/1  "xtof"
  OppOut.FrcCpl.Damper.xtof.x/1 -> OppOut.FrcCpl.Damper.xtof/1  "x"
  OppOut.FrcCpl.Damper.xtof.y/1 -> OppOut.FrcCpl.Damper.xtof/2  "y"
  OppOut.FrcCpl.Damper.xtof.z/1 -> OppOut.FrcCpl.Damper.xtof/3  "z"
  OppOut.FrcCpl.Damper.TransAx/1 -> OppOut.FrcCpl.Damper/2  "TransAx"
  OppOut.FrcCpl.Damper.TransAx.x/1 -> OppOut.FrcCpl.Damper.TransAx/1  "x"
  OppOut.FrcCpl.Damper.TransAx.y/1 -> OppOut.FrcCpl.Damper.TransAx/2  "y"
  OppOut.FrcCpl.Damper.TransAx.z/1 -> OppOut.FrcCpl.Damper.TransAx/3  "z"
  MainOut.Kin.ixtz/1 -> MainOut.Kin/3  "ixtz"
  MainOut.Kin.ixrz/1 -> MainOut.Kin/6  "ixrz"
  MainOut.Kin.ixSpring/1 -> MainOut.Kin/7  "ixSpring"
  MainOut.Kin.ixDamp/1 -> MainOut.Kin/8  "ixDamp"
  MainOut.Kin.ixBuf/1 -> MainOut.Kin/9  "ixBuf"
  MainOut.Kin.ixStabi/1 -> MainOut.Kin/10  "ixStabi"
  MainOut.dqComp.ixtz/1 -> MainOut.dqComp/3  "ixtz"
  MainOut.dqComp.ixSpring/1 -> MainOut.dqComp/7  "ixSpring"
  MainOut.dqComp.ixDamp/1 -> MainOut.dqComp/8  "ixDamp"
  MainOut.dqComp.ixBuf/1 -> MainOut.dqComp/9  "ixBuf"
  MainOut.dqComp.ixStabi/1 -> MainOut.dqComp/10  "ixStabi"
  MainOut.dqSteer.ixrz/1 -> MainOut.dqSteer/6  "ixrz"
  MainOut.Kin.ixtx/1 -> MainOut.Kin/1  "ixtx"
  MainOut.Kin.ixty/1 -> MainOut.Kin/2  "ixty"
  MainOut.Kin.ixrx/1 -> MainOut.Kin/4  "ixrx"
  MainOut.Kin.ixry/1 -> MainOut.Kin/5  "ixry"
  OppOut.Kin.ixtz/1 -> OppOut.Kin/3  "ixtz"
  OppOut.Kin.ixrz/1 -> OppOut.Kin/6  "ixrz"
  OppOut.Kin.ixSpring/1 -> OppOut.Kin/7  "ixSpring"
  OppOut.Kin.ixDamp/1 -> OppOut.Kin/8  "ixDamp"
  OppOut.Kin.ixBuf/1 -> OppOut.Kin/9  "ixBuf"
  OppOut.Kin.ixStabi/1 -> OppOut.Kin/10  "ixStabi"
  OppOut.dqComp.ixtz/1 -> OppOut.dqComp/3  "ixtz"
  OppOut.dqComp.ixSpring/1 -> OppOut.dqComp/7  "ixSpring"
  OppOut.dqComp.ixDamp/1 -> OppOut.dqComp/8  "ixDamp"
  OppOut.dqComp.ixBuf/1 -> OppOut.dqComp/9  "ixBuf"
  OppOut.dqComp.ixStabi/1 -> OppOut.dqComp/10  "ixStabi"
  OppOut.dqSteer.ixrz/1 -> OppOut.dqSteer/6  "ixrz"
